simulink model "1p_Full_ControlledConverter"  (R2020a)
settings: Solver=VariableStepAuto  StartTime=0.0  StopTime=0.1  RelTol=1e-3
libraries: powerlib x10, powerlib_meascontrol x2
settings Model: Creator=Siddharthan A  LastModifiedBy=Siddharthan A

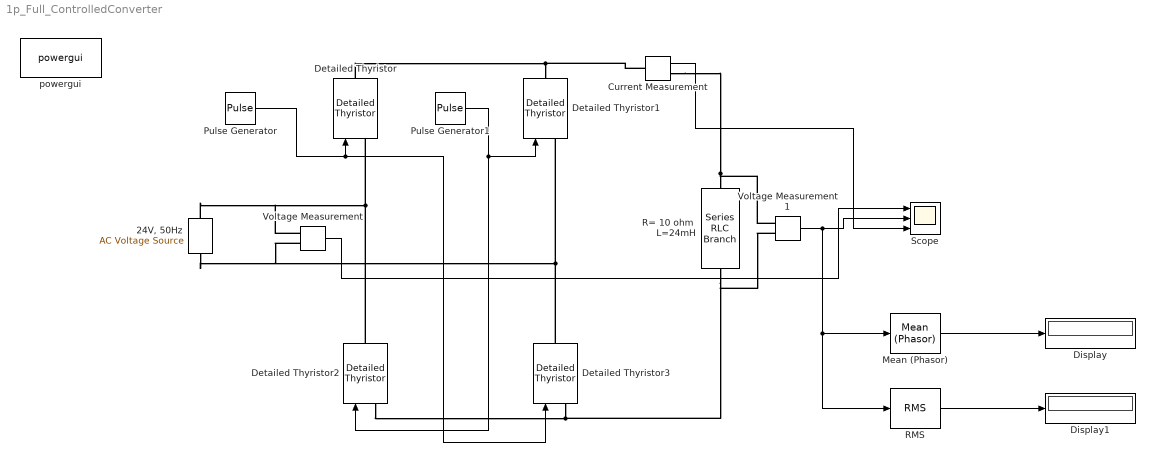
== system 1p_Full_ControlledConverter ==
  "24V, 50Hz" : powerlib/Electrical Sources/AC Voltage Source  Amplitude=24*sqrt(2)  Phase=0  Frequency=50  SampleTime=0  Measurements=None  BusType=swing  Pref=10e3  Qref=0  Qmin=-inf  Qmax=+inf
  Current Measurement : powerlib/Measurements/Current Measurement  PhasorSimulation=off  OutputType=Complex  PSBequivalent=0
  Detailed Thyristor{,1..3} (4 alike) : powerlib/Power Electronics/Detailed Thyristor  Ron=0.001  Lon=1e-3  Vf=0.8  IL=0.1  Tq=100e-6  IC=0  Rs=500  Cs=250e-9  Measurements=off
      settings: SourceProductBaseCode=PS
  Display : Display
  Display1 : Display
  Mean (Phasor) : powerlib_meascontrol/Measurements/Mean (Phasor)  Freq=60  Vinit=0  Ts=0
      settings: SourceProductBaseCode=PS
  Pulse Generator : DiscretePulseGenerator  PulseType=Time based  Period=0.02  PulseWidth=5  PhaseDelay=(0.01/pi)*(pi/4)
  Pulse Generator1 : DiscretePulseGenerator  PulseType=Time based  Period=0.02  PulseWidth=5  PhaseDelay=0.01+(0.01/pi)*(pi/4)
  R= 10 ohm  L=24mH : powerlib/Elements/Series RLC Branch  LConnTagsString=__new0  RConnTagsString=__new0  BranchType=R  Resistance=10  Inductance=24e-3  SetiL0=off  InitialCurrent=0  Capacitance=1e-6  Setx0=off  InitialVoltage=0  Measurements=None
  RMS : powerlib_meascontrol/Measurements/RMS  TrueRMS=on  Freq=60  RMSInit=120  Ts=0
  Scope : Scope  NumInputPorts=3
  Voltage Measurement : powerlib/Measurements/Voltage Measurement  PhasorSimulation=off  OutputType=Complex  PSBequivalent=0
  Voltage Measurement1 : powerlib/Measurements/Voltage Measurement  PhasorSimulation=off  OutputType=Complex  PSBequivalent=0
  powergui : powerlib/powergui  Priority=1  SimulationMode=Continuous  SampleTime=50e-6  frequency=60  Iterations=50  frequencyindice=50  Pbase=100e6  ErrMax=1e-4  UnitsV=kV  UnitsW=MW  buscounter=0  FunctionMessages=off  echomessages=off  EnableUseOfTLC=off  CurrentSourceSwitches=off  DisableSnubberDevices=off  DisableRonSwitches=off  DisableVfSwitches=off  DisplayEquations=off  AutomaticDiscreteSolvers=off  SolverType=Tustin/Backward Euler (TBE)  Interpol=off  ExternalGateDelay=off  methode=off  Ts=100  x0status=blocks  SPID=on  SwTol=0  HookPort=off  NonlinearTolerance=1e-4  nMaxIteration=100  ContinueOnMaxIteration=off  RestoreLinks=warning  ResistiveCurrentMeasurement=off  Frange=[0:2:500]  Ylog=off  Xlog=on  ShowGrid=off  save=off  variable=ZData  structure=0  ZoomFFT=off  StartTime=0.0  cycles=1  DisplayStyle=1  fundamental=60  FreqAxis=off  MaxFrequency=1000  frequencyindicesteady=1  RmsSteady=1  display=off
  wires:
  Voltage Measurement/1 -> Scope/1
  Voltage Measurement1/1 -> RMS/1, Mean (Phasor)/1, Scope/2
  Current Measurement/1 -> Scope/3
  Pulse Generator/1 -> Detailed Thyristor3/1, Detailed Thyristor/1
  Pulse Generator1/1 -> Detailed Thyristor2/1, Detailed Thyristor1/1
  Mean (Phasor)/1 -> Display/1
  RMS/1 -> Display1/1
  connections:
  Voltage Measurement/LConn1 -- "24V, 50Hz"/RConn1 -- Detailed Thyristor/LConn1 -- Detailed Thyristor2/RConn1
  Voltage Measurement/LConn2 -- "24V, 50Hz"/LConn1 -- Detailed Thyristor1/LConn1 -- Detailed Thyristor3/RConn1
  Detailed Thyristor/RConn1 -- Current Measurement/LConn1 -- Detailed Thyristor1/RConn1
  Voltage Measurement1/LConn2 -- R= 10 ohm  L=24mH/RConn1 -- Detailed Thyristor2/LConn1 -- Detailed Thyristor3/LConn1
  Current Measurement/RConn1 -- Voltage Measurement1/LConn1 -- R= 10 ohm  L=24mH/LConn1
